simulink model "modelosprimerasemana"  (R2023b)
settings: Solver=VariableStepAuto  StartTime=0.0  StopTime=10.0  RelTol=1e-3
libraries: arduinolib x3, simulink x1
settings Model: Creator=Pedro  LastModifiedBy=Pedro

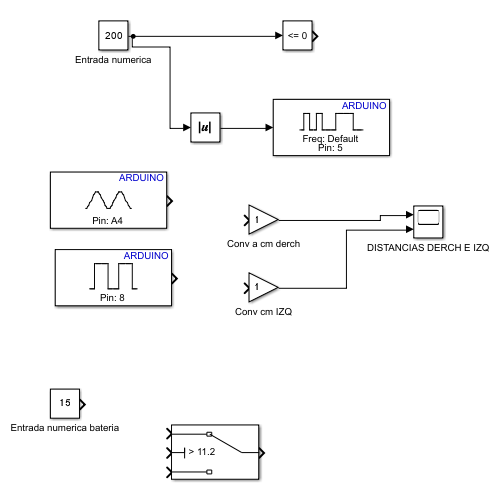
[thumbnail: Simulink's stored preview of the top-level diagram]
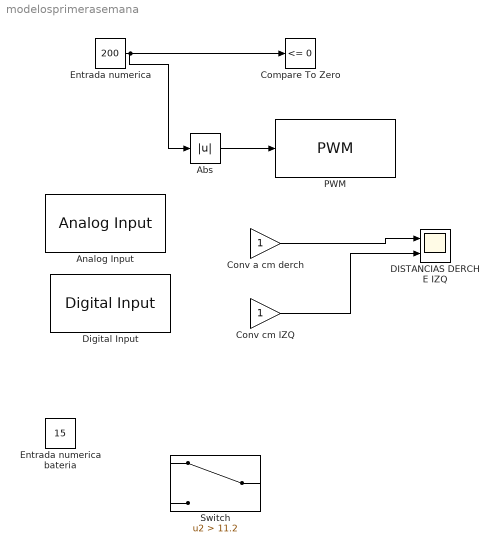
== system modelosprimerasemana ==
  Abs : Abs  SaturateOnIntegerOverflow=off
  Analog Input : arduinolib/Analog Input  pinNumber=4  ReadResultsOnly=off  ConversionTriggerSource=Software  ExternalTriggerType=uint32( 0 )  OutputDataType=uint16  EnableConversionCompleteNotify=off  EnableOuputStatus=off  SampleTime=-1  blockPlatform=arduino
  Compare To Zero : simulink/Logic and Bit Operations/Compare To Zero  relop=<=  OutDataTypeStr=boolean
  Conv a cm derch : Gain
  Conv cm IZQ : Gain
  DISTANCIAS DERCH E IZQ : Scope  NumInputPorts=2
  Digital Input : arduinolib/Digital Input  pinNumber=8  mode=Default  Direction=input  SampleTime=0.1  blockPlatform=arduino
  Entrada numerica : Constant  Value=200
  Entrada numerica bateria : Constant  Value=15
  PWM : arduinolib/PWM  pinNumber=5  frequencyType=Default  desiredFrequency=490.2  achievableFrequency=490.2
  Switch : Switch  Criteria=u2 > Threshold  Threshold=11.2  SaturateOnIntegerOverflow=off  InputSameDT=off
  wires:
  Entrada numerica/1 -> Abs/1, Compare To Zero/1
  Abs/1 -> PWM/1
  Conv a cm derch/1 -> DISTANCIAS DERCH E IZQ/1
  Conv cm IZQ/1 -> DISTANCIAS DERCH E IZQ/2
